simulink model "lab"  (R2021a)
settings: Solver=FixedStepAuto  StartTime=0.0  StopTime=10  FixedStep=1e-4  RelTol=1e-3
settings Model: Creator=rubro  LastModifiedBy=rubro

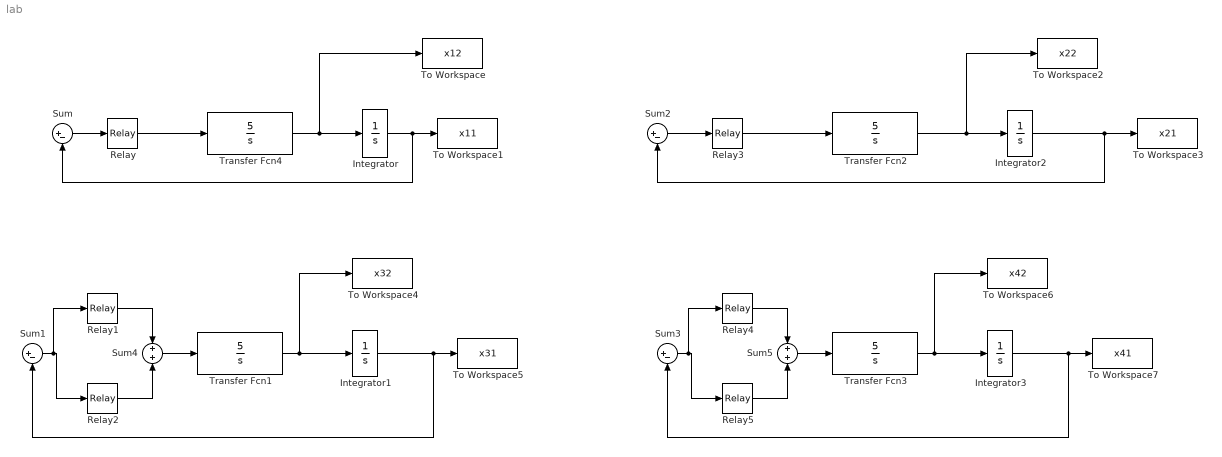
== system lab ==
  Integrator{,1..3} (4 alike) : Integrator  InitialCondition=1
  Relay : Relay  OnSwitchValue=0  OffSwitchValue=0  OffOutputValue=-1
  Relay1 : Relay  OnSwitchValue=0.1  OffSwitchValue=0.1
  Relay2 : Relay  OnSwitchValue=-0.1  OffSwitchValue=-0.1  OnOutputValue=0  OffOutputValue=-1
  Relay3 : Relay  OnSwitchValue=0.1  OffSwitchValue=-0.1  OffOutputValue=-1
  Relay4 : Relay  OnSwitchValue=-0.1  OffSwitchValue=-0.2  OnOutputValue=0  OffOutputValue=-1
  Relay5 : Relay  OnSwitchValue=0.2  OffSwitchValue=0.1
  Sum{,1..3} (4 alike) : Sum  Inputs=|+-
  Sum4 : Sum  Inputs=+|+
  Sum5 : Sum  Inputs=+|+
  To Workspace : ToWorkspace  VariableName=x12  SaveFormat=Structure  SampleTime=-1
  To Workspace1 : ToWorkspace  VariableName=x11  SaveFormat=Structure  SampleTime=-1
  To Workspace2 : ToWorkspace  VariableName=x22  SaveFormat=Structure  SampleTime=-1
  To Workspace3 : ToWorkspace  VariableName=x21  SaveFormat=Structure  SampleTime=-1
  To Workspace4 : ToWorkspace  VariableName=x32  SaveFormat=Structure  SampleTime=-1
  To Workspace5 : ToWorkspace  VariableName=x31  SaveFormat=Structure  SampleTime=-1
  To Workspace6 : ToWorkspace  VariableName=x42  SaveFormat=Structure  SampleTime=-1
      settings: Save2DSignal=2-D array (concatenate along first dimension)
  To Workspace7 : ToWorkspace  VariableName=x41  SaveFormat=Structure  SampleTime=-1
      settings: Save2DSignal=2-D array (concatenate along first dimension)
  Transfer Fcn1 : TransferFcn  Numerator=[5]  Denominator=[0 1 0]
  Transfer Fcn2 : TransferFcn  Numerator=[5]  Denominator=[0 1 0]
  Transfer Fcn3 : TransferFcn  Numerator=[5]  Denominator=[0 1 0]
  Transfer Fcn4 : TransferFcn  Numerator=[5]  Denominator=[1 0]
  wires:
  Sum1/1 -> Relay1/1, Relay2/1
  Transfer Fcn2/1 -> Integrator2/1, To Workspace2/1
  Integrator/1 -> Sum/2, To Workspace1/1
  Relay3/1 -> Transfer Fcn2/1
  Relay2/1 -> Sum4/2
  Transfer Fcn1/1 -> Integrator1/1, To Workspace4/1
  Relay1/1 -> Sum4/1
  Sum4/1 -> Transfer Fcn1/1
  Sum/1 -> Relay/1
  Sum2/1 -> Relay3/1
  Integrator2/1 -> To Workspace3/1, Sum2/2
  Transfer Fcn4/1 -> To Workspace/1, Integrator/1
  Relay/1 -> Transfer Fcn4/1
  Integrator1/1 -> Sum1/2, To Workspace5/1
  Integrator3/1 -> To Workspace7/1, Sum3/2
  Sum5/1 -> Transfer Fcn3/1
  Relay4/1 -> Sum5/1
  Transfer Fcn3/1 -> To Workspace6/1, Integrator3/1
  Relay5/1 -> Sum5/2
  Sum3/1 -> Relay5/1, Relay4/1
